simulink model "fec_ber_hw_V2"  (R2020b)
settings: Solver=FixedStepDiscrete  StartTime=0.0  StopTime=T  RelTol=1e-3
values from neighbouring files (symbols this model uses):
  aximm_awgn_reset = 0    [setup.m]
  aximm_bit_count_reset = 0    [setup.m]
  aximm_bits = n_blocks * k    (= 80)    [setup.m]
  aximm_ctrl_word_dec = 0    [setup.m]
  aximm_ctrl_word_enc = 0    [setup.m]
  aximm_enable = 1    [setup.m]
  aximm_length = k * n_blocks    (= 80)    [setup.m]
  aximm_length_dec = n    (= 160)    [setup.m]
  aximm_length_enc = k    (= 80)    [setup.m]
  aximm_llr_mag_reset = 0    [setup.m]
  aximm_llr_scale = (1/noise_var) * llr_scale    (= 1000)    [setup.m]
  aximm_load_dec = 1    [setup.m]
  aximm_load_enc = 1    [setup.m]
  aximm_noise_std = sqrt(noise_var)    [setup.m]
  aximm_reset = 0    [setup.m]
  d = sqrt(-2*log([0:1/4095:1]))    [setup.m]
  fs = 160e6    (= 160000000)    [setup.m]
  generator_polynomial = '''z^13 + z^12 + z^11 + z^8 + 1'''    [setup.m]
  llr_scale = 7.75/7.75    (= 1)    [setup.m]
libraries: simulink x931, hdlsllib x419, commseqgen3 x52, dspsigops x22, commblkcod2 x3, lib_rfsoc_fec x2
(part 33 of 47)

== system fec_ber_hw_V2/Soft Demodulation/SSR Soft Demodulation Lane 4/Soft Demodulation 5/Subsystem1 ==
  a : Inport
  b : Inport  Port=2
  a1 : Inport  Port=3
  b1 : Inport  Port=4
  a2 : Inport  Port=5
  b2 : Inport  Port=6
  a3 : Inport  Port=7
  b3 : Inport  Port=8
  get_min1 : Subsystem
  get_min2 : Subsystem
  get_min3 : Subsystem
  get_min4 : Subsystem
  get_min5 : Subsystem
  get_min6 : Subsystem
  get_min7 : Subsystem
  min : Outport
  wires:
  get_min5/1(min) -> get_min7/1(a)
  b2/1 -> get_min3/2(b)
  a/1 -> get_min1/1(a)
  get_min6/1(min) -> get_min7/2(b)
  get_min3/1(min) -> get_min6/1(a)
  b1/1 -> get_min2/2(b)
  get_min2/1(min) -> get_min5/2(b)
  get_min4/1(min) -> get_min6/2(b)
  a3/1 -> get_min4/1(a)
  get_min1/1(min) -> get_min5/1(a)
  get_min7/1(min) -> min/1
  b3/1 -> get_min4/2(b)
  a1/1 -> get_min2/1(a)
  b/1 -> get_min1/2(b)
  a2/1 -> get_min3/1(a)

== system fec_ber_hw_V2/Soft Demodulation/SSR Soft Demodulation Lane 4/Soft Demodulation 5/Subsystem2 ==
  a : Inport
  b : Inport  Port=2
  a1 : Inport  Port=3
  b1 : Inport  Port=4
  a2 : Inport  Port=5
  b2 : Inport  Port=6
  a3 : Inport  Port=7
  b3 : Inport  Port=8
  get_min1 : Subsystem
  get_min2 : Subsystem
  get_min3 : Subsystem
  get_min4 : Subsystem
  get_min5 : Subsystem
  get_min6 : Subsystem
  get_min7 : Subsystem
  min : Outport
  wires:
  get_min5/1(min) -> get_min7/1(a)
  b2/1 -> get_min3/2(b)
  a/1 -> get_min1/1(a)
  get_min6/1(min) -> get_min7/2(b)
  get_min3/1(min) -> get_min6/1(a)
  b1/1 -> get_min2/2(b)
  get_min2/1(min) -> get_min5/2(b)
  get_min4/1(min) -> get_min6/2(b)
  a3/1 -> get_min4/1(a)
  get_min1/1(min) -> get_min5/1(a)
  get_min7/1(min) -> min/1
  b3/1 -> get_min4/2(b)
  a1/1 -> get_min2/1(a)
  b/1 -> get_min1/2(b)
  a2/1 -> get_min3/1(a)

== system fec_ber_hw_V2/Soft Demodulation/SSR Soft Demodulation Lane 4/Soft Demodulation 5/Subsystem3 ==
  enb : Inport
  1-D Lookup Table : Lookup_n-D  NumberOfTableDimensions=1  BreakpointsForDimension1=[0:3]  IndexSearchMethod=Evenly spaced points  Table=z_y(1:8:end)  InterpMethod=Flat  DiagnosticForOutOfRangeInput=Error  InternalRulePriority=Speed  OutDataTypeStr=fixdt(1,3,0)  RndMeth=Simplest  InputSameDT=on
  1-D Lookup Table1 : Lookup_n-D  NumberOfTableDimensions=1  BreakpointsForDimension1=[0:3]  IndexSearchMethod=Evenly spaced points  Table=z_y(2:8:end)  InterpMethod=Flat  DiagnosticForOutOfRangeInput=Error  InternalRulePriority=Speed  OutDataTypeStr=fixdt(1,3,0)  RndMeth=Simplest  InputSameDT=on
  1-D Lookup Table2 : Lookup_n-D  NumberOfTableDimensions=1  BreakpointsForDimension1=[0:3]  IndexSearchMethod=Evenly spaced points  Table=z_y(3:8:end)  InterpMethod=Flat  DiagnosticForOutOfRangeInput=Error  InternalRulePriority=Speed  OutDataTypeStr=fixdt(1,3,0)  RndMeth=Simplest  InputSameDT=on
  1-D Lookup Table3 : Lookup_n-D  NumberOfTableDimensions=1  BreakpointsForDimension1=[0:3]  IndexSearchMethod=Evenly spaced points  Table=z_y(4:8:end)  InterpMethod=Flat  DiagnosticForOutOfRangeInput=Error  InternalRulePriority=Speed  OutDataTypeStr=fixdt(1,3,0)  RndMeth=Simplest  InputSameDT=on
  1-D Lookup Table4 : Lookup_n-D  NumberOfTableDimensions=1  BreakpointsForDimension1=[0:3]  IndexSearchMethod=Evenly spaced points  Table=z_y(5:8:end)  InterpMethod=Flat  DiagnosticForOutOfRangeInput=Error  InternalRulePriority=Speed  OutDataTypeStr=fixdt(1,3,0)  RndMeth=Simplest  InputSameDT=on
  1-D Lookup Table5 : Lookup_n-D  NumberOfTableDimensions=1  BreakpointsForDimension1=[0:3]  IndexSearchMethod=Evenly spaced points  Table=z_y(6:8:end)  InterpMethod=Flat  DiagnosticForOutOfRangeInput=Error  InternalRulePriority=Speed  OutDataTypeStr=fixdt(1,3,0)  RndMeth=Simplest  InputSameDT=on
  1-D Lookup Table6 : Lookup_n-D  NumberOfTableDimensions=1  BreakpointsForDimension1=[0:3]  IndexSearchMethod=Evenly spaced points  Table=z_y(7:8:end)  InterpMethod=Flat  DiagnosticForOutOfRangeInput=Error  InternalRulePriority=Speed  OutDataTypeStr=fixdt(1,3,0)  RndMeth=Simplest  InputSameDT=on
  1-D Lookup Table7 : Lookup_n-D  NumberOfTableDimensions=1  BreakpointsForDimension1=[0:3]  IndexSearchMethod=Evenly spaced points  Table=z_y(8:8:end)  InterpMethod=Flat  DiagnosticForOutOfRangeInput=Error  InternalRulePriority=Speed  OutDataTypeStr=fixdt(1,3,0)  RndMeth=Simplest  InputSameDT=on
  Out1 : Outport
  Out2 : Outport  Port=2
  Out3 : Outport  Port=3
  Out4 : Outport  Port=4
  Out5 : Outport  Port=5
  Out6 : Outport  Port=6
  Out7 : Outport  Port=7
  Out8 : Outport  Port=8
  wires:
  1-D Lookup Table6/1 -> Out7/1
  enb/1 -> 1-D Lookup Table4/1, 1-D Lookup Table5/1, 1-D Lookup Table6/1, 1-D Lookup Table7/1, 1-D Lookup Table/1, 1-D Lookup Table1/1, 1-D Lookup Table2/1, 1-D Lookup Table3/1
  1-D Lookup Table3/1 -> Out4/1
  1-D Lookup Table1/1 -> Out2/1
  1-D Lookup Table4/1 -> Out5/1
  1-D Lookup Table5/1 -> Out6/1
  1-D Lookup Table/1 -> Out1/1
  1-D Lookup Table2/1 -> Out3/1
  1-D Lookup Table7/1 -> Out8/1

== system fec_ber_hw_V2/Soft Demodulation/SSR Soft Demodulation Lane 4/Soft Demodulation 5/Subsystem4 ==
  enb : Inport
  1-D Lookup Table : Lookup_n-D  NumberOfTableDimensions=1  BreakpointsForDimension1=[0:3]  IndexSearchMethod=Evenly spaced points  Table=o_y(1:8:end)  InterpMethod=Flat  DiagnosticForOutOfRangeInput=Error  InternalRulePriority=Speed  OutDataTypeStr=fixdt(1,3,0)  RndMeth=Simplest  InputSameDT=on
  1-D Lookup Table1 : Lookup_n-D  NumberOfTableDimensions=1  BreakpointsForDimension1=[0:3]  IndexSearchMethod=Evenly spaced points  Table=o_y(2:8:end)  InterpMethod=Flat  DiagnosticForOutOfRangeInput=Error  InternalRulePriority=Speed  OutDataTypeStr=fixdt(1,3,0)  RndMeth=Simplest  InputSameDT=on
  1-D Lookup Table2 : Lookup_n-D  NumberOfTableDimensions=1  BreakpointsForDimension1=[0:3]  IndexSearchMethod=Evenly spaced points  Table=o_y(3:8:end)  InterpMethod=Flat  DiagnosticForOutOfRangeInput=Error  InternalRulePriority=Speed  OutDataTypeStr=fixdt(1,3,0)  RndMeth=Simplest  InputSameDT=on
  1-D Lookup Table3 : Lookup_n-D  NumberOfTableDimensions=1  BreakpointsForDimension1=[0:3]  IndexSearchMethod=Evenly spaced points  Table=o_y(4:8:end)  InterpMethod=Flat  DiagnosticForOutOfRangeInput=Error  InternalRulePriority=Speed  OutDataTypeStr=fixdt(1,3,0)  RndMeth=Simplest  InputSameDT=on
  1-D Lookup Table4 : Lookup_n-D  NumberOfTableDimensions=1  BreakpointsForDimension1=[0:3]  IndexSearchMethod=Evenly spaced points  Table=o_y(5:8:end)  InterpMethod=Flat  DiagnosticForOutOfRangeInput=Error  InternalRulePriority=Speed  OutDataTypeStr=fixdt(1,3,0)  RndMeth=Simplest  InputSameDT=on
  1-D Lookup Table5 : Lookup_n-D  NumberOfTableDimensions=1  BreakpointsForDimension1=[0:3]  IndexSearchMethod=Evenly spaced points  Table=o_y(6:8:end)  InterpMethod=Flat  DiagnosticForOutOfRangeInput=Error  InternalRulePriority=Speed  OutDataTypeStr=fixdt(1,3,0)  RndMeth=Simplest  InputSameDT=on
  1-D Lookup Table6 : Lookup_n-D  NumberOfTableDimensions=1  BreakpointsForDimension1=[0:3]  IndexSearchMethod=Evenly spaced points  Table=o_y(7:8:end)  InterpMethod=Flat  DiagnosticForOutOfRangeInput=Error  InternalRulePriority=Speed  OutDataTypeStr=fixdt(1,3,0)  RndMeth=Simplest  InputSameDT=on
  1-D Lookup Table7 : Lookup_n-D  NumberOfTableDimensions=1  BreakpointsForDimension1=[0:3]  IndexSearchMethod=Evenly spaced points  Table=o_y(8:8:end)  InterpMethod=Flat  DiagnosticForOutOfRangeInput=Error  InternalRulePriority=Speed  OutDataTypeStr=fixdt(1,3,0)  RndMeth=Simplest  InputSameDT=on
  Out1 : Outport
  Out2 : Outport  Port=2
  Out3 : Outport  Port=3
  Out4 : Outport  Port=4
  Out5 : Outport  Port=5
  Out6 : Outport  Port=6
  Out7 : Outport  Port=7
  Out8 : Outport  Port=8
  wires:
  1-D Lookup Table7/1 -> Out8/1
  1-D Lookup Table2/1 -> Out3/1
  1-D Lookup Table/1 -> Out1/1
  1-D Lookup Table5/1 -> Out6/1
  1-D Lookup Table4/1 -> Out5/1
  1-D Lookup Table1/1 -> Out2/1
  1-D Lookup Table3/1 -> Out4/1
  enb/1 -> 1-D Lookup Table7/1, 1-D Lookup Table6/1, 1-D Lookup Table5/1, 1-D Lookup Table4/1, 1-D Lookup Table3/1, 1-D Lookup Table2/1, 1-D Lookup Table1/1, 1-D Lookup Table/1
  1-D Lookup Table6/1 -> Out7/1

== system fec_ber_hw_V2/Soft Demodulation/SSR Soft Demodulation Lane 4/Soft Demodulation 5/Subsystem5 ==
  enb : Inport
  1-D Lookup Table : Lookup_n-D  NumberOfTableDimensions=1  BreakpointsForDimension1=[0:3]  IndexSearchMethod=Evenly spaced points  Table=o_x(1:8:end)  InterpMethod=Flat  DiagnosticForOutOfRangeInput=Error  InternalRulePriority=Speed  OutDataTypeStr=fixdt(1,3,0)  RndMeth=Simplest  InputSameDT=on
  1-D Lookup Table1 : Lookup_n-D  NumberOfTableDimensions=1  BreakpointsForDimension1=[0:3]  IndexSearchMethod=Evenly spaced points  Table=o_x(2:8:end)  InterpMethod=Flat  DiagnosticForOutOfRangeInput=Error  InternalRulePriority=Speed  OutDataTypeStr=fixdt(1,3,0)  RndMeth=Simplest  InputSameDT=on
  1-D Lookup Table2 : Lookup_n-D  NumberOfTableDimensions=1  BreakpointsForDimension1=[0:3]  IndexSearchMethod=Evenly spaced points  Table=o_x(3:8:end)  InterpMethod=Flat  DiagnosticForOutOfRangeInput=Error  InternalRulePriority=Speed  OutDataTypeStr=fixdt(1,3,0)  RndMeth=Simplest  InputSameDT=on
  1-D Lookup Table3 : Lookup_n-D  NumberOfTableDimensions=1  BreakpointsForDimension1=[0:3]  IndexSearchMethod=Evenly spaced points  Table=o_x(4:8:end)  InterpMethod=Flat  DiagnosticForOutOfRangeInput=Error  InternalRulePriority=Speed  OutDataTypeStr=fixdt(1,3,0)  RndMeth=Simplest  InputSameDT=on
  1-D Lookup Table4 : Lookup_n-D  NumberOfTableDimensions=1  BreakpointsForDimension1=[0:3]  IndexSearchMethod=Evenly spaced points  Table=o_x(5:8:end)  InterpMethod=Flat  DiagnosticForOutOfRangeInput=Error  InternalRulePriority=Speed  OutDataTypeStr=fixdt(1,3,0)  RndMeth=Simplest  InputSameDT=on
  1-D Lookup Table5 : Lookup_n-D  NumberOfTableDimensions=1  BreakpointsForDimension1=[0:3]  IndexSearchMethod=Evenly spaced points  Table=o_x(6:8:end)  InterpMethod=Flat  DiagnosticForOutOfRangeInput=Error  InternalRulePriority=Speed  OutDataTypeStr=fixdt(1,3,0)  RndMeth=Simplest  InputSameDT=on
  1-D Lookup Table6 : Lookup_n-D  NumberOfTableDimensions=1  BreakpointsForDimension1=[0:3]  IndexSearchMethod=Evenly spaced points  Table=o_x(7:8:end)  InterpMethod=Flat  DiagnosticForOutOfRangeInput=Error  InternalRulePriority=Speed  OutDataTypeStr=fixdt(1,3,0)  RndMeth=Simplest  InputSameDT=on
  1-D Lookup Table7 : Lookup_n-D  NumberOfTableDimensions=1  BreakpointsForDimension1=[0:3]  IndexSearchMethod=Evenly spaced points  Table=o_x(8:8:end)  InterpMethod=Flat  DiagnosticForOutOfRangeInput=Error  InternalRulePriority=Speed  OutDataTypeStr=fixdt(1,3,0)  RndMeth=Simplest  InputSameDT=on
  Out1 : Outport
  Out2 : Outport  Port=2
  Out3 : Outport  Port=3
  Out4 : Outport  Port=4
  Out5 : Outport  Port=5
  Out6 : Outport  Port=6
  Out7 : Outport  Port=7
  Out8 : Outport  Port=8
  wires:
  1-D Lookup Table6/1 -> Out7/1
  enb/1 -> 1-D Lookup Table/1, 1-D Lookup Table1/1, 1-D Lookup Table2/1, 1-D Lookup Table3/1, 1-D Lookup Table4/1, 1-D Lookup Table5/1, 1-D Lookup Table6/1, 1-D Lookup Table7/1
  1-D Lookup Table3/1 -> Out4/1
  1-D Lookup Table1/1 -> Out2/1
  1-D Lookup Table4/1 -> Out5/1
  1-D Lookup Table5/1 -> Out6/1
  1-D Lookup Table/1 -> Out1/1
  1-D Lookup Table2/1 -> Out3/1
  1-D Lookup Table7/1 -> Out8/1

== system fec_ber_hw_V2/Soft Demodulation/SSR Soft Demodulation Lane 4/Soft Demodulation 5/Subsystem6 ==
  enb : Inport
  1-D Lookup Table : Lookup_n-D  NumberOfTableDimensions=1  BreakpointsForDimension1=[0:3]  IndexSearchMethod=Evenly spaced points  Table=z_x(1:8:end)  InterpMethod=Flat  DiagnosticForOutOfRangeInput=Error  InternalRulePriority=Speed  OutDataTypeStr=fixdt(1,3,0)  RndMeth=Simplest  InputSameDT=on
  1-D Lookup Table1 : Lookup_n-D  NumberOfTableDimensions=1  BreakpointsForDimension1=[0:3]  IndexSearchMethod=Evenly spaced points  Table=z_x(2:8:end)  InterpMethod=Flat  DiagnosticForOutOfRangeInput=Error  InternalRulePriority=Speed  OutDataTypeStr=fixdt(1,3,0)  RndMeth=Simplest  InputSameDT=on
  1-D Lookup Table2 : Lookup_n-D  NumberOfTableDimensions=1  BreakpointsForDimension1=[0:3]  IndexSearchMethod=Evenly spaced points  Table=z_x(3:8:end)  InterpMethod=Flat  DiagnosticForOutOfRangeInput=Error  InternalRulePriority=Speed  OutDataTypeStr=fixdt(1,3,0)  RndMeth=Simplest  InputSameDT=on
  1-D Lookup Table3 : Lookup_n-D  NumberOfTableDimensions=1  BreakpointsForDimension1=[0:3]  IndexSearchMethod=Evenly spaced points  Table=z_x(4:8:end)  InterpMethod=Flat  DiagnosticForOutOfRangeInput=Error  InternalRulePriority=Speed  OutDataTypeStr=fixdt(1,3,0)  RndMeth=Simplest  InputSameDT=on
  1-D Lookup Table4 : Lookup_n-D  NumberOfTableDimensions=1  BreakpointsForDimension1=[0:3]  IndexSearchMethod=Evenly spaced points  Table=z_x(5:8:end)  InterpMethod=Flat  DiagnosticForOutOfRangeInput=Error  InternalRulePriority=Speed  OutDataTypeStr=fixdt(1,3,0)  RndMeth=Simplest  InputSameDT=on
  1-D Lookup Table5 : Lookup_n-D  NumberOfTableDimensions=1  BreakpointsForDimension1=[0:3]  IndexSearchMethod=Evenly spaced points  Table=z_x(6:8:end)  InterpMethod=Flat  DiagnosticForOutOfRangeInput=Error  InternalRulePriority=Speed  OutDataTypeStr=fixdt(1,3,0)  RndMeth=Simplest  InputSameDT=on
  1-D Lookup Table6 : Lookup_n-D  NumberOfTableDimensions=1  BreakpointsForDimension1=[0:3]  IndexSearchMethod=Evenly spaced points  Table=z_x(7:8:end)  InterpMethod=Flat  DiagnosticForOutOfRangeInput=Error  InternalRulePriority=Speed  OutDataTypeStr=fixdt(1,3,0)  RndMeth=Simplest  InputSameDT=on
  1-D Lookup Table7 : Lookup_n-D  NumberOfTableDimensions=1  BreakpointsForDimension1=[0:3]  IndexSearchMethod=Evenly spaced points  Table=z_x(8:8:end)  InterpMethod=Flat  DiagnosticForOutOfRangeInput=Error  InternalRulePriority=Speed  OutDataTypeStr=fixdt(1,3,0)  RndMeth=Simplest  InputSameDT=on
  Out1 : Outport
  Out2 : Outport  Port=2
  Out3 : Outport  Port=3
  Out4 : Outport  Port=4
  Out5 : Outport  Port=5
  Out6 : Outport  Port=6
  Out7 : Outport  Port=7
  Out8 : Outport  Port=8
  wires:
  1-D Lookup Table7/1 -> Out8/1
  1-D Lookup Table2/1 -> Out3/1
  1-D Lookup Table/1 -> Out1/1
  1-D Lookup Table5/1 -> Out6/1
  1-D Lookup Table4/1 -> Out5/1
  1-D Lookup Table1/1 -> Out2/1
  1-D Lookup Table3/1 -> Out4/1
  enb/1 -> 1-D Lookup Table3/1, 1-D Lookup Table2/1, 1-D Lookup Table1/1, 1-D Lookup Table/1, 1-D Lookup Table7/1, 1-D Lookup Table6/1, 1-D Lookup Table5/1, 1-D Lookup Table4/1
  1-D Lookup Table6/1 -> Out7/1

== system fec_ber_hw_V2/Soft Demodulation/SSR Soft Demodulation Lane 4/Soft Demodulation 5/sign_extend ==
  u : Inport
  Bit Concat : hdlsllib/Logic and Bit Operations/Bit Concat  numInputs=3
  Bit Slice : hdlsllib/Logic and Bit Operations/Bit Slice  lidx=5  ridx=5
      settings: SourceProductBaseCode=SL
  y : Outport
  wires:
  Bit Slice/1 -> Bit Concat/1, Bit Concat/2
  u/1 -> Bit Slice/1, Bit Concat/3
  Bit Concat/1 -> y/1

== system fec_ber_hw_V2/Soft Demodulation/SSR Soft Demodulation Lane 4/Soft Demodulation 6/Subsystem1 ==
  a : Inport
  b : Inport  Port=2
  a1 : Inport  Port=3
  b1 : Inport  Port=4
  a2 : Inport  Port=5
  b2 : Inport  Port=6
  a3 : Inport  Port=7
  b3 : Inport  Port=8
  get_min1 : Subsystem
  get_min2 : Subsystem
  get_min3 : Subsystem
  get_min4 : Subsystem
  get_min5 : Subsystem
  get_min6 : Subsystem
  get_min7 : Subsystem
  min : Outport
  wires:
  get_min5/1(min) -> get_min7/1(a)
  b2/1 -> get_min3/2(b)
  a/1 -> get_min1/1(a)
  get_min6/1(min) -> get_min7/2(b)
  get_min3/1(min) -> get_min6/1(a)
  b1/1 -> get_min2/2(b)
  get_min2/1(min) -> get_min5/2(b)
  get_min4/1(min) -> get_min6/2(b)
  a3/1 -> get_min4/1(a)
  get_min1/1(min) -> get_min5/1(a)
  get_min7/1(min) -> min/1
  b3/1 -> get_min4/2(b)
  a1/1 -> get_min2/1(a)
  b/1 -> get_min1/2(b)
  a2/1 -> get_min3/1(a)

== system fec_ber_hw_V2/Soft Demodulation/SSR Soft Demodulation Lane 4/Soft Demodulation 6/Subsystem2 ==
  a : Inport
  b : Inport  Port=2
  a1 : Inport  Port=3
  b1 : Inport  Port=4
  a2 : Inport  Port=5
  b2 : Inport  Port=6
  a3 : Inport  Port=7
  b3 : Inport  Port=8
  get_min1 : Subsystem
  get_min2 : Subsystem
  get_min3 : Subsystem
  get_min4 : Subsystem
  get_min5 : Subsystem
  get_min6 : Subsystem
  get_min7 : Subsystem
  min : Outport
  wires:
  get_min5/1(min) -> get_min7/1(a)
  b2/1 -> get_min3/2(b)
  a/1 -> get_min1/1(a)
  get_min6/1(min) -> get_min7/2(b)
  get_min3/1(min) -> get_min6/1(a)
  b1/1 -> get_min2/2(b)
  get_min2/1(min) -> get_min5/2(b)
  get_min4/1(min) -> get_min6/2(b)
  a3/1 -> get_min4/1(a)
  get_min1/1(min) -> get_min5/1(a)
  get_min7/1(min) -> min/1
  b3/1 -> get_min4/2(b)
  a1/1 -> get_min2/1(a)
  b/1 -> get_min1/2(b)
  a2/1 -> get_min3/1(a)

== system fec_ber_hw_V2/Soft Demodulation/SSR Soft Demodulation Lane 4/Soft Demodulation 6/Subsystem3 ==
  enb : Inport
  1-D Lookup Table : Lookup_n-D  NumberOfTableDimensions=1  BreakpointsForDimension1=[0:3]  IndexSearchMethod=Evenly spaced points  Table=z_y(1:8:end)  InterpMethod=Flat  DiagnosticForOutOfRangeInput=Error  InternalRulePriority=Speed  OutDataTypeStr=fixdt(1,3,0)  RndMeth=Simplest  InputSameDT=on
  1-D Lookup Table1 : Lookup_n-D  NumberOfTableDimensions=1  BreakpointsForDimension1=[0:3]  IndexSearchMethod=Evenly spaced points  Table=z_y(2:8:end)  InterpMethod=Flat  DiagnosticForOutOfRangeInput=Error  InternalRulePriority=Speed  OutDataTypeStr=fixdt(1,3,0)  RndMeth=Simplest  InputSameDT=on
  1-D Lookup Table2 : Lookup_n-D  NumberOfTableDimensions=1  BreakpointsForDimension1=[0:3]  IndexSearchMethod=Evenly spaced points  Table=z_y(3:8:end)  InterpMethod=Flat  DiagnosticForOutOfRangeInput=Error  InternalRulePriority=Speed  OutDataTypeStr=fixdt(1,3,0)  RndMeth=Simplest  InputSameDT=on
  1-D Lookup Table3 : Lookup_n-D  NumberOfTableDimensions=1  BreakpointsForDimension1=[0:3]  IndexSearchMethod=Evenly spaced points  Table=z_y(4:8:end)  InterpMethod=Flat  DiagnosticForOutOfRangeInput=Error  InternalRulePriority=Speed  OutDataTypeStr=fixdt(1,3,0)  RndMeth=Simplest  InputSameDT=on
  1-D Lookup Table4 : Lookup_n-D  NumberOfTableDimensions=1  BreakpointsForDimension1=[0:3]  IndexSearchMethod=Evenly spaced points  Table=z_y(5:8:end)  InterpMethod=Flat  DiagnosticForOutOfRangeInput=Error  InternalRulePriority=Speed  OutDataTypeStr=fixdt(1,3,0)  RndMeth=Simplest  InputSameDT=on
  1-D Lookup Table5 : Lookup_n-D  NumberOfTableDimensions=1  BreakpointsForDimension1=[0:3]  IndexSearchMethod=Evenly spaced points  Table=z_y(6:8:end)  InterpMethod=Flat  DiagnosticForOutOfRangeInput=Error  InternalRulePriority=Speed  OutDataTypeStr=fixdt(1,3,0)  RndMeth=Simplest  InputSameDT=on
  1-D Lookup Table6 : Lookup_n-D  NumberOfTableDimensions=1  BreakpointsForDimension1=[0:3]  IndexSearchMethod=Evenly spaced points  Table=z_y(7:8:end)  InterpMethod=Flat  DiagnosticForOutOfRangeInput=Error  InternalRulePriority=Speed  OutDataTypeStr=fixdt(1,3,0)  RndMeth=Simplest  InputSameDT=on
  1-D Lookup Table7 : Lookup_n-D  NumberOfTableDimensions=1  BreakpointsForDimension1=[0:3]  IndexSearchMethod=Evenly spaced points  Table=z_y(8:8:end)  InterpMethod=Flat  DiagnosticForOutOfRangeInput=Error  InternalRulePriority=Speed  OutDataTypeStr=fixdt(1,3,0)  RndMeth=Simplest  InputSameDT=on
  Out1 : Outport
  Out2 : Outport  Port=2
  Out3 : Outport  Port=3
  Out4 : Outport  Port=4
  Out5 : Outport  Port=5
  Out6 : Outport  Port=6
  Out7 : Outport  Port=7
  Out8 : Outport  Port=8
  wires:
  1-D Lookup Table6/1 -> Out7/1
  enb/1 -> 1-D Lookup Table4/1, 1-D Lookup Table5/1, 1-D Lookup Table6/1, 1-D Lookup Table7/1, 1-D Lookup Table/1, 1-D Lookup Table1/1, 1-D Lookup Table2/1, 1-D Lookup Table3/1
  1-D Lookup Table3/1 -> Out4/1
  1-D Lookup Table1/1 -> Out2/1
  1-D Lookup Table4/1 -> Out5/1
  1-D Lookup Table5/1 -> Out6/1
  1-D Lookup Table/1 -> Out1/1
  1-D Lookup Table2/1 -> Out3/1
  1-D Lookup Table7/1 -> Out8/1

== system fec_ber_hw_V2/Soft Demodulation/SSR Soft Demodulation Lane 4/Soft Demodulation 6/Subsystem4 ==
  enb : Inport
  1-D Lookup Table : Lookup_n-D  NumberOfTableDimensions=1  BreakpointsForDimension1=[0:3]  IndexSearchMethod=Evenly spaced points  Table=o_y(1:8:end)  InterpMethod=Flat  DiagnosticForOutOfRangeInput=Error  InternalRulePriority=Speed  OutDataTypeStr=fixdt(1,3,0)  RndMeth=Simplest  InputSameDT=on
  1-D Lookup Table1 : Lookup_n-D  NumberOfTableDimensions=1  BreakpointsForDimension1=[0:3]  IndexSearchMethod=Evenly spaced points  Table=o_y(2:8:end)  InterpMethod=Flat  DiagnosticForOutOfRangeInput=Error  InternalRulePriority=Speed  OutDataTypeStr=fixdt(1,3,0)  RndMeth=Simplest  InputSameDT=on
  1-D Lookup Table2 : Lookup_n-D  NumberOfTableDimensions=1  BreakpointsForDimension1=[0:3]  IndexSearchMethod=Evenly spaced points  Table=o_y(3:8:end)  InterpMethod=Flat  DiagnosticForOutOfRangeInput=Error  InternalRulePriority=Speed  OutDataTypeStr=fixdt(1,3,0)  RndMeth=Simplest  InputSameDT=on
  1-D Lookup Table3 : Lookup_n-D  NumberOfTableDimensions=1  BreakpointsForDimension1=[0:3]  IndexSearchMethod=Evenly spaced points  Table=o_y(4:8:end)  InterpMethod=Flat  DiagnosticForOutOfRangeInput=Error  InternalRulePriority=Speed  OutDataTypeStr=fixdt(1,3,0)  RndMeth=Simplest  InputSameDT=on
  1-D Lookup Table4 : Lookup_n-D  NumberOfTableDimensions=1  BreakpointsForDimension1=[0:3]  IndexSearchMethod=Evenly spaced points  Table=o_y(5:8:end)  InterpMethod=Flat  DiagnosticForOutOfRangeInput=Error  InternalRulePriority=Speed  OutDataTypeStr=fixdt(1,3,0)  RndMeth=Simplest  InputSameDT=on
  1-D Lookup Table5 : Lookup_n-D  NumberOfTableDimensions=1  BreakpointsForDimension1=[0:3]  IndexSearchMethod=Evenly spaced points  Table=o_y(6:8:end)  InterpMethod=Flat  DiagnosticForOutOfRangeInput=Error  InternalRulePriority=Speed  OutDataTypeStr=fixdt(1,3,0)  RndMeth=Simplest  InputSameDT=on
  1-D Lookup Table6 : Lookup_n-D  NumberOfTableDimensions=1  BreakpointsForDimension1=[0:3]  IndexSearchMethod=Evenly spaced points  Table=o_y(7:8:end)  InterpMethod=Flat  DiagnosticForOutOfRangeInput=Error  InternalRulePriority=Speed  OutDataTypeStr=fixdt(1,3,0)  RndMeth=Simplest  InputSameDT=on
  1-D Lookup Table7 : Lookup_n-D  NumberOfTableDimensions=1  BreakpointsForDimension1=[0:3]  IndexSearchMethod=Evenly spaced points  Table=o_y(8:8:end)  InterpMethod=Flat  DiagnosticForOutOfRangeInput=Error  InternalRulePriority=Speed  OutDataTypeStr=fixdt(1,3,0)  RndMeth=Simplest  InputSameDT=on
  Out1 : Outport
  Out2 : Outport  Port=2
  Out3 : Outport  Port=3
  Out4 : Outport  Port=4
  Out5 : Outport  Port=5
  Out6 : Outport  Port=6
  Out7 : Outport  Port=7
  Out8 : Outport  Port=8
  wires:
  1-D Lookup Table7/1 -> Out8/1
  1-D Lookup Table2/1 -> Out3/1
  1-D Lookup Table/1 -> Out1/1
  1-D Lookup Table5/1 -> Out6/1
  1-D Lookup Table4/1 -> Out5/1
  1-D Lookup Table1/1 -> Out2/1
  1-D Lookup Table3/1 -> Out4/1
  enb/1 -> 1-D Lookup Table7/1, 1-D Lookup Table6/1, 1-D Lookup Table5/1, 1-D Lookup Table4/1, 1-D Lookup Table3/1, 1-D Lookup Table2/1, 1-D Lookup Table1/1, 1-D Lookup Table/1
  1-D Lookup Table6/1 -> Out7/1

== system fec_ber_hw_V2/Soft Demodulation/SSR Soft Demodulation Lane 4/Soft Demodulation 6/Subsystem5 ==
  enb : Inport
  1-D Lookup Table : Lookup_n-D  NumberOfTableDimensions=1  BreakpointsForDimension1=[0:3]  IndexSearchMethod=Evenly spaced points  Table=o_x(1:8:end)  InterpMethod=Flat  DiagnosticForOutOfRangeInput=Error  InternalRulePriority=Speed  OutDataTypeStr=fixdt(1,3,0)  RndMeth=Simplest  InputSameDT=on
  1-D Lookup Table1 : Lookup_n-D  NumberOfTableDimensions=1  BreakpointsForDimension1=[0:3]  IndexSearchMethod=Evenly spaced points  Table=o_x(2:8:end)  InterpMethod=Flat  DiagnosticForOutOfRangeInput=Error  InternalRulePriority=Speed  OutDataTypeStr=fixdt(1,3,0)  RndMeth=Simplest  InputSameDT=on
  1-D Lookup Table2 : Lookup_n-D  NumberOfTableDimensions=1  BreakpointsForDimension1=[0:3]  IndexSearchMethod=Evenly spaced points  Table=o_x(3:8:end)  InterpMethod=Flat  DiagnosticForOutOfRangeInput=Error  InternalRulePriority=Speed  OutDataTypeStr=fixdt(1,3,0)  RndMeth=Simplest  InputSameDT=on
  1-D Lookup Table3 : Lookup_n-D  NumberOfTableDimensions=1  BreakpointsForDimension1=[0:3]  IndexSearchMethod=Evenly spaced points  Table=o_x(4:8:end)  InterpMethod=Flat  DiagnosticForOutOfRangeInput=Error  InternalRulePriority=Speed  OutDataTypeStr=fixdt(1,3,0)  RndMeth=Simplest  InputSameDT=on
  1-D Lookup Table4 : Lookup_n-D  NumberOfTableDimensions=1  BreakpointsForDimension1=[0:3]  IndexSearchMethod=Evenly spaced points  Table=o_x(5:8:end)  InterpMethod=Flat  DiagnosticForOutOfRangeInput=Error  InternalRulePriority=Speed  OutDataTypeStr=fixdt(1,3,0)  RndMeth=Simplest  InputSameDT=on
  1-D Lookup Table5 : Lookup_n-D  NumberOfTableDimensions=1  BreakpointsForDimension1=[0:3]  IndexSearchMethod=Evenly spaced points  Table=o_x(6:8:end)  InterpMethod=Flat  DiagnosticForOutOfRangeInput=Error  InternalRulePriority=Speed  OutDataTypeStr=fixdt(1,3,0)  RndMeth=Simplest  InputSameDT=on
  1-D Lookup Table6 : Lookup_n-D  NumberOfTableDimensions=1  BreakpointsForDimension1=[0:3]  IndexSearchMethod=Evenly spaced points  Table=o_x(7:8:end)  InterpMethod=Flat  DiagnosticForOutOfRangeInput=Error  InternalRulePriority=Speed  OutDataTypeStr=fixdt(1,3,0)  RndMeth=Simplest  InputSameDT=on
  1-D Lookup Table7 : Lookup_n-D  NumberOfTableDimensions=1  BreakpointsForDimension1=[0:3]  IndexSearchMethod=Evenly spaced points  Table=o_x(8:8:end)  InterpMethod=Flat  DiagnosticForOutOfRangeInput=Error  InternalRulePriority=Speed  OutDataTypeStr=fixdt(1,3,0)  RndMeth=Simplest  InputSameDT=on
  Out1 : Outport
  Out2 : Outport  Port=2
  Out3 : Outport  Port=3
  Out4 : Outport  Port=4
  Out5 : Outport  Port=5
  Out6 : Outport  Port=6
  Out7 : Outport  Port=7
  Out8 : Outport  Port=8
  wires:
  1-D Lookup Table6/1 -> Out7/1
  enb/1 -> 1-D Lookup Table/1, 1-D Lookup Table1/1, 1-D Lookup Table2/1, 1-D Lookup Table3/1, 1-D Lookup Table4/1, 1-D Lookup Table5/1, 1-D Lookup Table6/1, 1-D Lookup Table7/1
  1-D Lookup Table3/1 -> Out4/1
  1-D Lookup Table1/1 -> Out2/1
  1-D Lookup Table4/1 -> Out5/1
  1-D Lookup Table5/1 -> Out6/1
  1-D Lookup Table/1 -> Out1/1
  1-D Lookup Table2/1 -> Out3/1
  1-D Lookup Table7/1 -> Out8/1

== system fec_ber_hw_V2/Soft Demodulation/SSR Soft Demodulation Lane 4/Soft Demodulation 6/Subsystem6 ==
  enb : Inport
  1-D Lookup Table : Lookup_n-D  NumberOfTableDimensions=1  BreakpointsForDimension1=[0:3]  IndexSearchMethod=Evenly spaced points  Table=z_x(1:8:end)  InterpMethod=Flat  DiagnosticForOutOfRangeInput=Error  InternalRulePriority=Speed  OutDataTypeStr=fixdt(1,3,0)  RndMeth=Simplest  InputSameDT=on
  1-D Lookup Table1 : Lookup_n-D  NumberOfTableDimensions=1  BreakpointsForDimension1=[0:3]  IndexSearchMethod=Evenly spaced points  Table=z_x(2:8:end)  InterpMethod=Flat  DiagnosticForOutOfRangeInput=Error  InternalRulePriority=Speed  OutDataTypeStr=fixdt(1,3,0)  RndMeth=Simplest  InputSameDT=on
  1-D Lookup Table2 : Lookup_n-D  NumberOfTableDimensions=1  BreakpointsForDimension1=[0:3]  IndexSearchMethod=Evenly spaced points  Table=z_x(3:8:end)  InterpMethod=Flat  DiagnosticForOutOfRangeInput=Error  InternalRulePriority=Speed  OutDataTypeStr=fixdt(1,3,0)  RndMeth=Simplest  InputSameDT=on
  1-D Lookup Table3 : Lookup_n-D  NumberOfTableDimensions=1  BreakpointsForDimension1=[0:3]  IndexSearchMethod=Evenly spaced points  Table=z_x(4:8:end)  InterpMethod=Flat  DiagnosticForOutOfRangeInput=Error  InternalRulePriority=Speed  OutDataTypeStr=fixdt(1,3,0)  RndMeth=Simplest  InputSameDT=on
  1-D Lookup Table4 : Lookup_n-D  NumberOfTableDimensions=1  BreakpointsForDimension1=[0:3]  IndexSearchMethod=Evenly spaced points  Table=z_x(5:8:end)  InterpMethod=Flat  DiagnosticForOutOfRangeInput=Error  InternalRulePriority=Speed  OutDataTypeStr=fixdt(1,3,0)  RndMeth=Simplest  InputSameDT=on
  1-D Lookup Table5 : Lookup_n-D  NumberOfTableDimensions=1  BreakpointsForDimension1=[0:3]  IndexSearchMethod=Evenly spaced points  Table=z_x(6:8:end)  InterpMethod=Flat  DiagnosticForOutOfRangeInput=Error  InternalRulePriority=Speed  OutDataTypeStr=fixdt(1,3,0)  RndMeth=Simplest  InputSameDT=on
  1-D Lookup Table6 : Lookup_n-D  NumberOfTableDimensions=1  BreakpointsForDimension1=[0:3]  IndexSearchMethod=Evenly spaced points  Table=z_x(7:8:end)  InterpMethod=Flat  DiagnosticForOutOfRangeInput=Error  InternalRulePriority=Speed  OutDataTypeStr=fixdt(1,3,0)  RndMeth=Simplest  InputSameDT=on
  1-D Lookup Table7 : Lookup_n-D  NumberOfTableDimensions=1  BreakpointsForDimension1=[0:3]  IndexSearchMethod=Evenly spaced points  Table=z_x(8:8:end)  InterpMethod=Flat  DiagnosticForOutOfRangeInput=Error  InternalRulePriority=Speed  OutDataTypeStr=fixdt(1,3,0)  RndMeth=Simplest  InputSameDT=on
  Out1 : Outport
  Out2 : Outport  Port=2
  Out3 : Outport  Port=3
  Out4 : Outport  Port=4
  Out5 : Outport  Port=5
  Out6 : Outport  Port=6
  Out7 : Outport  Port=7
  Out8 : Outport  Port=8
  wires:
  1-D Lookup Table7/1 -> Out8/1
  1-D Lookup Table2/1 -> Out3/1
  1-D Lookup Table/1 -> Out1/1
  1-D Lookup Table5/1 -> Out6/1
  1-D Lookup Table4/1 -> Out5/1
  1-D Lookup Table1/1 -> Out2/1
  1-D Lookup Table3/1 -> Out4/1
  enb/1 -> 1-D Lookup Table3/1, 1-D Lookup Table2/1, 1-D Lookup Table1/1, 1-D Lookup Table/1, 1-D Lookup Table7/1, 1-D Lookup Table6/1, 1-D Lookup Table5/1, 1-D Lookup Table4/1
  1-D Lookup Table6/1 -> Out7/1

== system fec_ber_hw_V2/Soft Demodulation/SSR Soft Demodulation Lane 4/Soft Demodulation 6/sign_extend ==
  u : Inport
  Bit Concat : hdlsllib/Logic and Bit Operations/Bit Concat  numInputs=3
  Bit Slice : hdlsllib/Logic and Bit Operations/Bit Slice  lidx=5  ridx=5
      settings: SourceProductBaseCode=SL
  y : Outport
  wires:
  Bit Slice/1 -> Bit Concat/1, Bit Concat/2
  u/1 -> Bit Slice/1, Bit Concat/3
  Bit Concat/1 -> y/1

== system fec_ber_hw_V2/Soft Demodulation/SSR Soft Demodulation Lane 4/Soft Demodulation 7/Subsystem1 ==
  a : Inport
  b : Inport  Port=2
  a1 : Inport  Port=3
  b1 : Inport  Port=4
  a2 : Inport  Port=5
  b2 : Inport  Port=6
  a3 : Inport  Port=7
  b3 : Inport  Port=8
  get_min1 : Subsystem
  get_min2 : Subsystem
  get_min3 : Subsystem
  get_min4 : Subsystem
  get_min5 : Subsystem
  get_min6 : Subsystem
  get_min7 : Subsystem
  min : Outport
  wires:
  get_min5/1(min) -> get_min7/1(a)
  b2/1 -> get_min3/2(b)
  a/1 -> get_min1/1(a)
  get_min6/1(min) -> get_min7/2(b)
  get_min3/1(min) -> get_min6/1(a)
  b1/1 -> get_min2/2(b)
  get_min2/1(min) -> get_min5/2(b)
  get_min4/1(min) -> get_min6/2(b)
  a3/1 -> get_min4/1(a)
  get_min1/1(min) -> get_min5/1(a)
  get_min7/1(min) -> min/1
  b3/1 -> get_min4/2(b)
  a1/1 -> get_min2/1(a)
  b/1 -> get_min1/2(b)
  a2/1 -> get_min3/1(a)

== system fec_ber_hw_V2/Soft Demodulation/SSR Soft Demodulation Lane 4/Soft Demodulation 7/Subsystem2 ==
  a : Inport
  b : Inport  Port=2
  a1 : Inport  Port=3
  b1 : Inport  Port=4
  a2 : Inport  Port=5
  b2 : Inport  Port=6
  a3 : Inport  Port=7
  b3 : Inport  Port=8
  get_min1 : Subsystem
  get_min2 : Subsystem
  get_min3 : Subsystem
  get_min4 : Subsystem
  get_min5 : Subsystem
  get_min6 : Subsystem
  get_min7 : Subsystem
  min : Outport
  wires:
  get_min5/1(min) -> get_min7/1(a)
  b2/1 -> get_min3/2(b)
  a/1 -> get_min1/1(a)
  get_min6/1(min) -> get_min7/2(b)
  get_min3/1(min) -> get_min6/1(a)
  b1/1 -> get_min2/2(b)
  get_min2/1(min) -> get_min5/2(b)
  get_min4/1(min) -> get_min6/2(b)
  a3/1 -> get_min4/1(a)
  get_min1/1(min) -> get_min5/1(a)
  get_min7/1(min) -> min/1
  b3/1 -> get_min4/2(b)
  a1/1 -> get_min2/1(a)
  b/1 -> get_min1/2(b)
  a2/1 -> get_min3/1(a)

== system fec_ber_hw_V2/Soft Demodulation/SSR Soft Demodulation Lane 4/Soft Demodulation 7/Subsystem3 ==
  enb : Inport
  1-D Lookup Table : Lookup_n-D  NumberOfTableDimensions=1  BreakpointsForDimension1=[0:3]  IndexSearchMethod=Evenly spaced points  Table=z_y(1:8:end)  InterpMethod=Flat  DiagnosticForOutOfRangeInput=Error  InternalRulePriority=Speed  OutDataTypeStr=fixdt(1,3,0)  RndMeth=Simplest  InputSameDT=on
  1-D Lookup Table1 : Lookup_n-D  NumberOfTableDimensions=1  BreakpointsForDimension1=[0:3]  IndexSearchMethod=Evenly spaced points  Table=z_y(2:8:end)  InterpMethod=Flat  DiagnosticForOutOfRangeInput=Error  InternalRulePriority=Speed  OutDataTypeStr=fixdt(1,3,0)  RndMeth=Simplest  InputSameDT=on
  1-D Lookup Table2 : Lookup_n-D  NumberOfTableDimensions=1  BreakpointsForDimension1=[0:3]  IndexSearchMethod=Evenly spaced points  Table=z_y(3:8:end)  InterpMethod=Flat  DiagnosticForOutOfRangeInput=Error  InternalRulePriority=Speed  OutDataTypeStr=fixdt(1,3,0)  RndMeth=Simplest  InputSameDT=on
  1-D Lookup Table3 : Lookup_n-D  NumberOfTableDimensions=1  BreakpointsForDimension1=[0:3]  IndexSearchMethod=Evenly spaced points  Table=z_y(4:8:end)  InterpMethod=Flat  DiagnosticForOutOfRangeInput=Error  InternalRulePriority=Speed  OutDataTypeStr=fixdt(1,3,0)  RndMeth=Simplest  InputSameDT=on
  1-D Lookup Table4 : Lookup_n-D  NumberOfTableDimensions=1  BreakpointsForDimension1=[0:3]  IndexSearchMethod=Evenly spaced points  Table=z_y(5:8:end)  InterpMethod=Flat  DiagnosticForOutOfRangeInput=Error  InternalRulePriority=Speed  OutDataTypeStr=fixdt(1,3,0)  RndMeth=Simplest  InputSameDT=on
  1-D Lookup Table5 : Lookup_n-D  NumberOfTableDimensions=1  BreakpointsForDimension1=[0:3]  IndexSearchMethod=Evenly spaced points  Table=z_y(6:8:end)  InterpMethod=Flat  DiagnosticForOutOfRangeInput=Error  InternalRulePriority=Speed  OutDataTypeStr=fixdt(1,3,0)  RndMeth=Simplest  InputSameDT=on
  1-D Lookup Table6 : Lookup_n-D  NumberOfTableDimensions=1  BreakpointsForDimension1=[0:3]  IndexSearchMethod=Evenly spaced points  Table=z_y(7:8:end)  InterpMethod=Flat  DiagnosticForOutOfRangeInput=Error  InternalRulePriority=Speed  OutDataTypeStr=fixdt(1,3,0)  RndMeth=Simplest  InputSameDT=on
  1-D Lookup Table7 : Lookup_n-D  NumberOfTableDimensions=1  BreakpointsForDimension1=[0:3]  IndexSearchMethod=Evenly spaced points  Table=z_y(8:8:end)  InterpMethod=Flat  DiagnosticForOutOfRangeInput=Error  InternalRulePriority=Speed  OutDataTypeStr=fixdt(1,3,0)  RndMeth=Simplest  InputSameDT=on
  Out1 : Outport
  Out2 : Outport  Port=2
  Out3 : Outport  Port=3
  Out4 : Outport  Port=4
  Out5 : Outport  Port=5
  Out6 : Outport  Port=6
  Out7 : Outport  Port=7
  Out8 : Outport  Port=8
  wires:
  1-D Lookup Table6/1 -> Out7/1
  enb/1 -> 1-D Lookup Table4/1, 1-D Lookup Table5/1, 1-D Lookup Table6/1, 1-D Lookup Table7/1, 1-D Lookup Table/1, 1-D Lookup Table1/1, 1-D Lookup Table2/1, 1-D Lookup Table3/1
  1-D Lookup Table3/1 -> Out4/1
  1-D Lookup Table1/1 -> Out2/1
  1-D Lookup Table4/1 -> Out5/1
  1-D Lookup Table5/1 -> Out6/1
  1-D Lookup Table/1 -> Out1/1
  1-D Lookup Table2/1 -> Out3/1
  1-D Lookup Table7/1 -> Out8/1

== system fec_ber_hw_V2/Soft Demodulation/SSR Soft Demodulation Lane 4/Soft Demodulation 7/Subsystem4 ==
  enb : Inport
  1-D Lookup Table : Lookup_n-D  NumberOfTableDimensions=1  BreakpointsForDimension1=[0:3]  IndexSearchMethod=Evenly spaced points  Table=o_y(1:8:end)  InterpMethod=Flat  DiagnosticForOutOfRangeInput=Error  InternalRulePriority=Speed  OutDataTypeStr=fixdt(1,3,0)  RndMeth=Simplest  InputSameDT=on
  1-D Lookup Table1 : Lookup_n-D  NumberOfTableDimensions=1  BreakpointsForDimension1=[0:3]  IndexSearchMethod=Evenly spaced points  Table=o_y(2:8:end)  InterpMethod=Flat  DiagnosticForOutOfRangeInput=Error  InternalRulePriority=Speed  OutDataTypeStr=fixdt(1,3,0)  RndMeth=Simplest  InputSameDT=on
  1-D Lookup Table2 : Lookup_n-D  NumberOfTableDimensions=1  BreakpointsForDimension1=[0:3]  IndexSearchMethod=Evenly spaced points  Table=o_y(3:8:end)  InterpMethod=Flat  DiagnosticForOutOfRangeInput=Error  InternalRulePriority=Speed  OutDataTypeStr=fixdt(1,3,0)  RndMeth=Simplest  InputSameDT=on
  1-D Lookup Table3 : Lookup_n-D  NumberOfTableDimensions=1  BreakpointsForDimension1=[0:3]  IndexSearchMethod=Evenly spaced points  Table=o_y(4:8:end)  InterpMethod=Flat  DiagnosticForOutOfRangeInput=Error  InternalRulePriority=Speed  OutDataTypeStr=fixdt(1,3,0)  RndMeth=Simplest  InputSameDT=on
  1-D Lookup Table4 : Lookup_n-D  NumberOfTableDimensions=1  BreakpointsForDimension1=[0:3]  IndexSearchMethod=Evenly spaced points  Table=o_y(5:8:end)  InterpMethod=Flat  DiagnosticForOutOfRangeInput=Error  InternalRulePriority=Speed  OutDataTypeStr=fixdt(1,3,0)  RndMeth=Simplest  InputSameDT=on
  1-D Lookup Table5 : Lookup_n-D  NumberOfTableDimensions=1  BreakpointsForDimension1=[0:3]  IndexSearchMethod=Evenly spaced points  Table=o_y(6:8:end)  InterpMethod=Flat  DiagnosticForOutOfRangeInput=Error  InternalRulePriority=Speed  OutDataTypeStr=fixdt(1,3,0)  RndMeth=Simplest  InputSameDT=on
  1-D Lookup Table6 : Lookup_n-D  NumberOfTableDimensions=1  BreakpointsForDimension1=[0:3]  IndexSearchMethod=Evenly spaced points  Table=o_y(7:8:end)  InterpMethod=Flat  DiagnosticForOutOfRangeInput=Error  InternalRulePriority=Speed  OutDataTypeStr=fixdt(1,3,0)  RndMeth=Simplest  InputSameDT=on
  1-D Lookup Table7 : Lookup_n-D  NumberOfTableDimensions=1  BreakpointsForDimension1=[0:3]  IndexSearchMethod=Evenly spaced points  Table=o_y(8:8:end)  InterpMethod=Flat  DiagnosticForOutOfRangeInput=Error  InternalRulePriority=Speed  OutDataTypeStr=fixdt(1,3,0)  RndMeth=Simplest  InputSameDT=on
  Out1 : Outport
  Out2 : Outport  Port=2
  Out3 : Outport  Port=3
  Out4 : Outport  Port=4
  Out5 : Outport  Port=5
  Out6 : Outport  Port=6
  Out7 : Outport  Port=7
  Out8 : Outport  Port=8
  wires:
  1-D Lookup Table7/1 -> Out8/1
  1-D Lookup Table2/1 -> Out3/1
  1-D Lookup Table/1 -> Out1/1
  1-D Lookup Table5/1 -> Out6/1
  1-D Lookup Table4/1 -> Out5/1
  1-D Lookup Table1/1 -> Out2/1
  1-D Lookup Table3/1 -> Out4/1
  enb/1 -> 1-D Lookup Table7/1, 1-D Lookup Table6/1, 1-D Lookup Table5/1, 1-D Lookup Table4/1, 1-D Lookup Table3/1, 1-D Lookup Table2/1, 1-D Lookup Table1/1, 1-D Lookup Table/1
  1-D Lookup Table6/1 -> Out7/1

== system fec_ber_hw_V2/Soft Demodulation/SSR Soft Demodulation Lane 4/Soft Demodulation 7/Subsystem5 ==
  enb : Inport
  1-D Lookup Table : Lookup_n-D  NumberOfTableDimensions=1  BreakpointsForDimension1=[0:3]  IndexSearchMethod=Evenly spaced points  Table=o_x(1:8:end)  InterpMethod=Flat  DiagnosticForOutOfRangeInput=Error  InternalRulePriority=Speed  OutDataTypeStr=fixdt(1,3,0)  RndMeth=Simplest  InputSameDT=on
  1-D Lookup Table1 : Lookup_n-D  NumberOfTableDimensions=1  BreakpointsForDimension1=[0:3]  IndexSearchMethod=Evenly spaced points  Table=o_x(2:8:end)  InterpMethod=Flat  DiagnosticForOutOfRangeInput=Error  InternalRulePriority=Speed  OutDataTypeStr=fixdt(1,3,0)  RndMeth=Simplest  InputSameDT=on
  1-D Lookup Table2 : Lookup_n-D  NumberOfTableDimensions=1  BreakpointsForDimension1=[0:3]  IndexSearchMethod=Evenly spaced points  Table=o_x(3:8:end)  InterpMethod=Flat  DiagnosticForOutOfRangeInput=Error  InternalRulePriority=Speed  OutDataTypeStr=fixdt(1,3,0)  RndMeth=Simplest  InputSameDT=on
  1-D Lookup Table3 : Lookup_n-D  NumberOfTableDimensions=1  BreakpointsForDimension1=[0:3]  IndexSearchMethod=Evenly spaced points  Table=o_x(4:8:end)  InterpMethod=Flat  DiagnosticForOutOfRangeInput=Error  InternalRulePriority=Speed  OutDataTypeStr=fixdt(1,3,0)  RndMeth=Simplest  InputSameDT=on
  1-D Lookup Table4 : Lookup_n-D  NumberOfTableDimensions=1  BreakpointsForDimension1=[0:3]  IndexSearchMethod=Evenly spaced points  Table=o_x(5:8:end)  InterpMethod=Flat  DiagnosticForOutOfRangeInput=Error  InternalRulePriority=Speed  OutDataTypeStr=fixdt(1,3,0)  RndMeth=Simplest  InputSameDT=on
  1-D Lookup Table5 : Lookup_n-D  NumberOfTableDimensions=1  BreakpointsForDimension1=[0:3]  IndexSearchMethod=Evenly spaced points  Table=o_x(6:8:end)  InterpMethod=Flat  DiagnosticForOutOfRangeInput=Error  InternalRulePriority=Speed  OutDataTypeStr=fixdt(1,3,0)  RndMeth=Simplest  InputSameDT=on
  1-D Lookup Table6 : Lookup_n-D  NumberOfTableDimensions=1  BreakpointsForDimension1=[0:3]  IndexSearchMethod=Evenly spaced points  Table=o_x(7:8:end)  InterpMethod=Flat  DiagnosticForOutOfRangeInput=Error  InternalRulePriority=Speed  OutDataTypeStr=fixdt(1,3,0)  RndMeth=Simplest  InputSameDT=on
  1-D Lookup Table7 : Lookup_n-D  NumberOfTableDimensions=1  BreakpointsForDimension1=[0:3]  IndexSearchMethod=Evenly spaced points  Table=o_x(8:8:end)  InterpMethod=Flat  DiagnosticForOutOfRangeInput=Error  InternalRulePriority=Speed  OutDataTypeStr=fixdt(1,3,0)  RndMeth=Simplest  InputSameDT=on
  Out1 : Outport
  Out2 : Outport  Port=2
  Out3 : Outport  Port=3
  Out4 : Outport  Port=4
  Out5 : Outport  Port=5
  Out6 : Outport  Port=6
  Out7 : Outport  Port=7
  Out8 : Outport  Port=8
  wires:
  1-D Lookup Table6/1 -> Out7/1
  enb/1 -> 1-D Lookup Table/1, 1-D Lookup Table1/1, 1-D Lookup Table2/1, 1-D Lookup Table3/1, 1-D Lookup Table4/1, 1-D Lookup Table5/1, 1-D Lookup Table6/1, 1-D Lookup Table7/1
  1-D Lookup Table3/1 -> Out4/1
  1-D Lookup Table1/1 -> Out2/1
  1-D Lookup Table4/1 -> Out5/1
  1-D Lookup Table5/1 -> Out6/1
  1-D Lookup Table/1 -> Out1/1
  1-D Lookup Table2/1 -> Out3/1
  1-D Lookup Table7/1 -> Out8/1

== system fec_ber_hw_V2/Soft Demodulation/SSR Soft Demodulation Lane 4/Soft Demodulation 7/Subsystem6 ==
  enb : Inport
  1-D Lookup Table : Lookup_n-D  NumberOfTableDimensions=1  BreakpointsForDimension1=[0:3]  IndexSearchMethod=Evenly spaced points  Table=z_x(1:8:end)  InterpMethod=Flat  DiagnosticForOutOfRangeInput=Error  InternalRulePriority=Speed  OutDataTypeStr=fixdt(1,3,0)  RndMeth=Simplest  InputSameDT=on
  1-D Lookup Table1 : Lookup_n-D  NumberOfTableDimensions=1  BreakpointsForDimension1=[0:3]  IndexSearchMethod=Evenly spaced points  Table=z_x(2:8:end)  InterpMethod=Flat  DiagnosticForOutOfRangeInput=Error  InternalRulePriority=Speed  OutDataTypeStr=fixdt(1,3,0)  RndMeth=Simplest  InputSameDT=on
  1-D Lookup Table2 : Lookup_n-D  NumberOfTableDimensions=1  BreakpointsForDimension1=[0:3]  IndexSearchMethod=Evenly spaced points  Table=z_x(3:8:end)  InterpMethod=Flat  DiagnosticForOutOfRangeInput=Error  InternalRulePriority=Speed  OutDataTypeStr=fixdt(1,3,0)  RndMeth=Simplest  InputSameDT=on
  1-D Lookup Table3 : Lookup_n-D  NumberOfTableDimensions=1  BreakpointsForDimension1=[0:3]  IndexSearchMethod=Evenly spaced points  Table=z_x(4:8:end)  InterpMethod=Flat  DiagnosticForOutOfRangeInput=Error  InternalRulePriority=Speed  OutDataTypeStr=fixdt(1,3,0)  RndMeth=Simplest  InputSameDT=on
  1-D Lookup Table4 : Lookup_n-D  NumberOfTableDimensions=1  BreakpointsForDimension1=[0:3]  IndexSearchMethod=Evenly spaced points  Table=z_x(5:8:end)  InterpMethod=Flat  DiagnosticForOutOfRangeInput=Error  InternalRulePriority=Speed  OutDataTypeStr=fixdt(1,3,0)  RndMeth=Simplest  InputSameDT=on
  1-D Lookup Table5 : Lookup_n-D  NumberOfTableDimensions=1  BreakpointsForDimension1=[0:3]  IndexSearchMethod=Evenly spaced points  Table=z_x(6:8:end)  InterpMethod=Flat  DiagnosticForOutOfRangeInput=Error  InternalRulePriority=Speed  OutDataTypeStr=fixdt(1,3,0)  RndMeth=Simplest  InputSameDT=on
  1-D Lookup Table6 : Lookup_n-D  NumberOfTableDimensions=1  BreakpointsForDimension1=[0:3]  IndexSearchMethod=Evenly spaced points  Table=z_x(7:8:end)  InterpMethod=Flat  DiagnosticForOutOfRangeInput=Error  InternalRulePriority=Speed  OutDataTypeStr=fixdt(1,3,0)  RndMeth=Simplest  InputSameDT=on
  1-D Lookup Table7 : Lookup_n-D  NumberOfTableDimensions=1  BreakpointsForDimension1=[0:3]  IndexSearchMethod=Evenly spaced points  Table=z_x(8:8:end)  InterpMethod=Flat  DiagnosticForOutOfRangeInput=Error  InternalRulePriority=Speed  OutDataTypeStr=fixdt(1,3,0)  RndMeth=Simplest  InputSameDT=on
  Out1 : Outport
  Out2 : Outport  Port=2
  Out3 : Outport  Port=3
  Out4 : Outport  Port=4
  Out5 : Outport  Port=5
  Out6 : Outport  Port=6
  Out7 : Outport  Port=7
  Out8 : Outport  Port=8
  wires:
  1-D Lookup Table7/1 -> Out8/1
  1-D Lookup Table2/1 -> Out3/1
  1-D Lookup Table/1 -> Out1/1
  1-D Lookup Table5/1 -> Out6/1
  1-D Lookup Table4/1 -> Out5/1
  1-D Lookup Table1/1 -> Out2/1
  1-D Lookup Table3/1 -> Out4/1
  enb/1 -> 1-D Lookup Table3/1, 1-D Lookup Table2/1, 1-D Lookup Table1/1, 1-D Lookup Table/1, 1-D Lookup Table7/1, 1-D Lookup Table6/1, 1-D Lookup Table5/1, 1-D Lookup Table4/1
  1-D Lookup Table6/1 -> Out7/1

== system fec_ber_hw_V2/Soft Demodulation/SSR Soft Demodulation Lane 4/Soft Demodulation 7/sign_extend ==
  u : Inport
  Bit Concat : hdlsllib/Logic and Bit Operations/Bit Concat  numInputs=3
  Bit Slice : hdlsllib/Logic and Bit Operations/Bit Slice  lidx=5  ridx=5
      settings: SourceProductBaseCode=SL
  y : Outport
  wires:
  Bit Slice/1 -> Bit Concat/1, Bit Concat/2
  u/1 -> Bit Slice/1, Bit Concat/3
  Bit Concat/1 -> y/1

== system fec_ber_hw_V2/Soft Demodulation1/Soft Demodulation 0/Subsystem1/get_min1 ==
  a : Inport
  b : Inport  Port=2
  Compare To Zero : simulink/Logic and Bit Operations/Compare To Zero  relop=<=  OutDataTypeStr=boolean
  Multiport Switch2 : MultiPortSwitch  DataPortOrder=Zero-based contiguous  Inputs=2  zeroidx=on
  Subtract18 : Sum  Inputs=+-  OutDataTypeStr=fixdt(1,(w+1)*2+2,f*2)  SaturateOnIntegerOverflow=on
  min : Outport
  wires:
  Subtract18/1 -> Compare To Zero/1
  b/1 -> Subtract18/2, Multiport Switch2/2
  a/1 -> Multiport Switch2/3, Subtract18/1
  Multiport Switch2/1 -> min/1
  Compare To Zero/1 -> Multiport Switch2/1

== system fec_ber_hw_V2/Soft Demodulation1/Soft Demodulation 0/Subsystem1/get_min2 ==
  a : Inport
  b : Inport  Port=2
  Compare To Zero : simulink/Logic and Bit Operations/Compare To Zero  relop=<=  OutDataTypeStr=boolean
  Multiport Switch2 : MultiPortSwitch  DataPortOrder=Zero-based contiguous  Inputs=2  zeroidx=on
  Subtract18 : Sum  Inputs=+-  OutDataTypeStr=fixdt(1,(w+1)*2+2,f*2)  SaturateOnIntegerOverflow=on
  min : Outport
  wires:
  Compare To Zero/1 -> Multiport Switch2/1
  Multiport Switch2/1 -> min/1
  a/1 -> Subtract18/1, Multiport Switch2/3
  b/1 -> Multiport Switch2/2, Subtract18/2
  Subtract18/1 -> Compare To Zero/1

== system fec_ber_hw_V2/Soft Demodulation1/Soft Demodulation 0/Subsystem1/get_min3 ==
  a : Inport
  b : Inport  Port=2
  Compare To Zero : simulink/Logic and Bit Operations/Compare To Zero  relop=<=  OutDataTypeStr=boolean
  Multiport Switch2 : MultiPortSwitch  DataPortOrder=Zero-based contiguous  Inputs=2  zeroidx=on
  Subtract18 : Sum  Inputs=+-  OutDataTypeStr=fixdt(1,(w+1)*2+2,f*2)  SaturateOnIntegerOverflow=on
  min : Outport
  wires:
  Subtract18/1 -> Compare To Zero/1
  b/1 -> Subtract18/2, Multiport Switch2/2
  a/1 -> Multiport Switch2/3, Subtract18/1
  Multiport Switch2/1 -> min/1
  Compare To Zero/1 -> Multiport Switch2/1

== system fec_ber_hw_V2/Soft Demodulation1/Soft Demodulation 0/Subsystem1/get_min4 ==
  a : Inport
  b : Inport  Port=2
  Compare To Zero : simulink/Logic and Bit Operations/Compare To Zero  relop=<=  OutDataTypeStr=boolean
  Multiport Switch2 : MultiPortSwitch  DataPortOrder=Zero-based contiguous  Inputs=2  zeroidx=on
  Subtract18 : Sum  Inputs=+-  OutDataTypeStr=fixdt(1,(w+1)*2+2,f*2)  SaturateOnIntegerOverflow=on
  min : Outport
  wires:
  Compare To Zero/1 -> Multiport Switch2/1
  Multiport Switch2/1 -> min/1
  a/1 -> Subtract18/1, Multiport Switch2/3
  b/1 -> Multiport Switch2/2, Subtract18/2
  Subtract18/1 -> Compare To Zero/1

== system fec_ber_hw_V2/Soft Demodulation1/Soft Demodulation 0/Subsystem1/get_min5 ==
  a : Inport
  b : Inport  Port=2
  Compare To Zero : simulink/Logic and Bit Operations/Compare To Zero  relop=<=  OutDataTypeStr=boolean
  Multiport Switch2 : MultiPortSwitch  DataPortOrder=Zero-based contiguous  Inputs=2  zeroidx=on
  Subtract18 : Sum  Inputs=+-  OutDataTypeStr=fixdt(1,(w+1)*2+2,f*2)  SaturateOnIntegerOverflow=on
  min : Outport
  wires:
  Subtract18/1 -> Compare To Zero/1
  b/1 -> Subtract18/2, Multiport Switch2/2
  a/1 -> Multiport Switch2/3, Subtract18/1
  Multiport Switch2/1 -> min/1
  Compare To Zero/1 -> Multiport Switch2/1

== system fec_ber_hw_V2/Soft Demodulation1/Soft Demodulation 0/Subsystem1/get_min6 ==
  a : Inport
  b : Inport  Port=2
  Compare To Zero : simulink/Logic and Bit Operations/Compare To Zero  relop=<=  OutDataTypeStr=boolean
  Multiport Switch2 : MultiPortSwitch  DataPortOrder=Zero-based contiguous  Inputs=2  zeroidx=on
  Subtract18 : Sum  Inputs=+-  OutDataTypeStr=fixdt(1,(w+1)*2+2,f*2)  SaturateOnIntegerOverflow=on
  min : Outport
  wires:
  Compare To Zero/1 -> Multiport Switch2/1
  Multiport Switch2/1 -> min/1
  a/1 -> Subtract18/1, Multiport Switch2/3
  b/1 -> Multiport Switch2/2, Subtract18/2
  Subtract18/1 -> Compare To Zero/1
